simulink model "mpc_demo"  (R2016b)
settings: Solver=ode45  StartTime=0.0  StopTime=20.0  MaxStep=0.01  RelTol=1e-3  EnableMultiTasking=on
undefined symbols (not defined in the file): DiscIntNeverNeededParam
libraries: simulink x1
settings Model: Creator=jgillis  LastModifiedBy=z041288
settings DataIOCC: LimitDataPoints=on  SaveFormat=Array
settings OptimizationCC: LifeSpan=inf
settings DebuggingCC: SolverPrmCheckMsg=warning  SFUnexpectedBacktrackingDiag=warning  SFNoUnconditionalDefaultTransitionDiag=warning  SFExecutionAtInitializationDiag=none
settings HardwareCC: ProdBitPerPointer=32  ProdBitPerSizeT=32  ProdBitPerPtrDiffT=32  ProdLargestAtomicFloat=None  ProdIntDivRoundTo=Undefined  ProdEndianess=Unspecified  ProdWordSize=32  ProdHWDeviceType=32-bit Generic
settings ModelReferenceCC: PropagateSignalLabelsOutOfModel=off
settings GRTTargetCC: TargetLangStandard=C89/C90 (ANSI)  GeneratePreprocessorConditionals=Disable all
settings ConfigComp: CovMetricSettings=dw  CovHtmlReporting=on  CovSaveCumulativeToWorkspaceVar=on  CovSaveSingleToWorkspaceVar=on  CovExternalEMLEnable=off  CovSFcnEnable=off

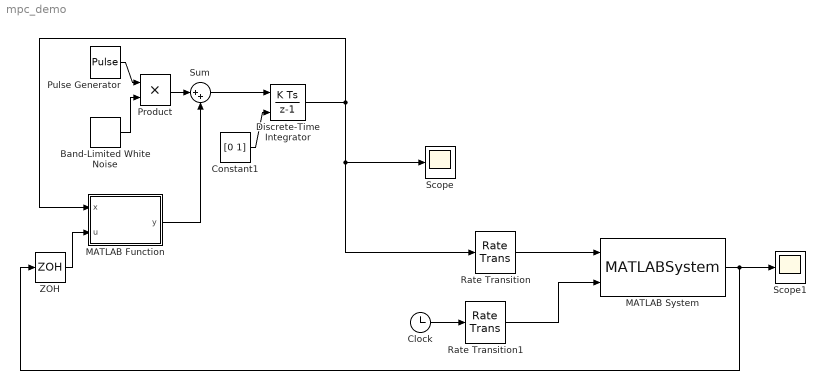
== system mpc_demo ==
  Band-Limited White Noise : simulink/Sources/Band-Limited White Noise  Cov=[1]  Ts=0.1  seed=[23341]
  Clock : Clock
  Constant1 : Constant  Value=[0 1]
  Discrete-Time Integrator : DiscreteIntegrator  InitialConditionSource=external  InitialConditionSetting=State (most efficient)  SampleTime=-1  ICPrevOutput=DiscIntNeverNeededParam  ICPrevScaledInput=DiscIntNeverNeededParam
  MATLAB Function : MATLAB Function  TreatAsAtomicUnit=on
  MATLAB System : MATLABSystem  System=casadi_block  SimulateUsing=Interpreted execution
      mask Type: casadi_block
      mask Display:
      | disp('casadi_block');
      | port_label('input',1,'x');
      | port_label('input',2,'t');
      | port_label('output',1,'u');
  Product : Product
  Pulse Generator : DiscretePulseGenerator  PulseType=Time based  Period=10  PulseWidth=5  PhaseDelay=10
  Rate Transition : RateTransition  OutPortSampleTime=0.1
  Rate Transition1 : RateTransition  OutPortSampleTime=0.1
  Scope : Scope
  Scope1 : Scope
  Sum : Sum  Inputs=|++
  ZOH : ZeroOrderHold  SampleTime=0.1
  wires:
  MATLAB Function/1(y) -> Sum/2
  Discrete-Time Integrator/1 -> MATLAB Function/1(x), Rate Transition/1, Scope/1
  Constant1/1 -> Discrete-Time Integrator/2
  MATLAB System/1 -> Scope1/1, ZOH/1
  ZOH/1 -> MATLAB Function/2(u)
  Clock/1 -> Rate Transition1/1
  Rate Transition/1 -> MATLAB System/1
  Rate Transition1/1 -> MATLAB System/2
  Sum/1 -> Discrete-Time Integrator/1
  Band-Limited White Noise/1 -> Product/2
  Product/1 -> Sum/1
  Pulse Generator/1 -> Product/1

== matlab function mpc_demo/MATLAB Function ==
  data: x input; u input; y output
function y = rhs(x,u)
%#codegen

y = [(1-x(2)^2)*x(1) - x(2) + u; x(1)];


end
